simulink model "xyzFuzzyQuadControl"  (R2014b)
settings: Solver=ode45  StartTime=0.0  StopTime=100  RelTol=1e-3
values from neighbouring files (symbols this model uses):
  b = 3.13e-5    (= 3.13e-05)    [Parrametresnnlineaire.m]
  d = 7.50e-7    (= 7.5e-07)    [Parrametresnnlineaire.m]
  g = 9.81    [Parrametresnnlineaire.m]
  Ix = 0.0075    [Parrametresnnlineaire.m]
  Iy = 0.0075    [Parrametresnnlineaire.m]
  Iz = 0.013    [Parrametresnnlineaire.m]
  Jr = 6e-5    (= 6e-05)    [Parrametresnnlineaire.m]
  l = 0.23    [Parrametresnnlineaire.m]
  m = 0.65    [Parrametresnnlineaire.m]
undefined symbols (not defined in the file or in its folder): sigbuilder_block
libraries: fuzblock x6, simulink x5
settings Model: Creator=Khadija  LastModifiedBy=Khadija
settings DataIOCC: LimitDataPoints=off

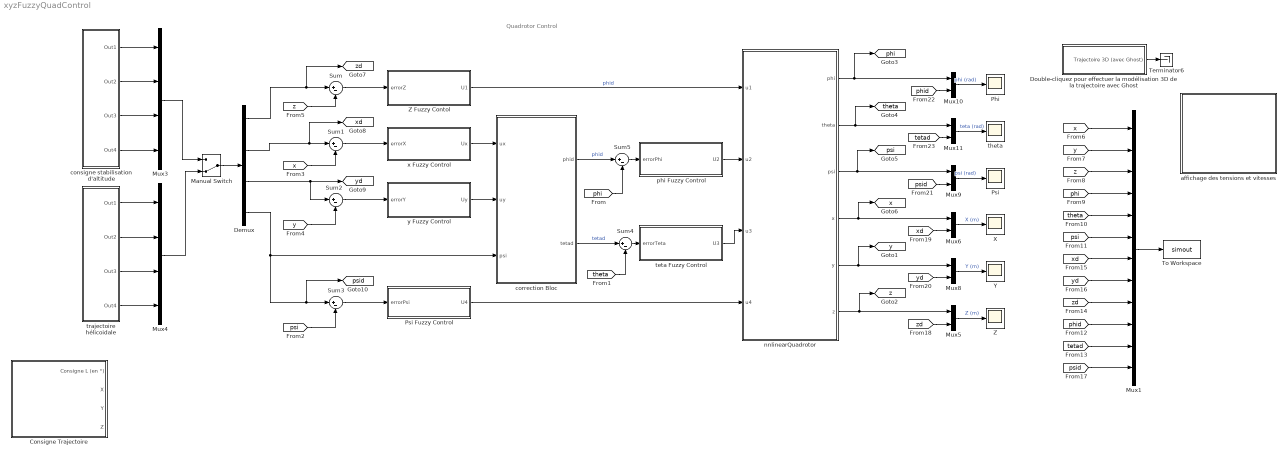
== system xyzFuzzyQuadControl ==
  note: Quadrotor Control
  " Z Fuzzy Contol" : Subsystem
  " phi Fuzzy Control " : Subsystem
  " x Fuzzy Control " : Subsystem
  Consigne Trajectoire : Subsystem  Tag=STV Subsys  LoadFcn=sigbuilder_block('load');  StartFcn=sigbuilder_block('start');  StopFcn=sigbuilder_block('stop');  ClipboardFcn=sigbuilder_block('clipboard');  mask(Sigbuilder block){}
      mask help: Sigbuilder GUI
      mask init:
      | if ~strcmp(get_param(bdroot(gcbh),'SimulationStatus'),'stopped') tuvar = sigbuilder_block('maskInit'); end
      settings: CopyFcn=sigbuilder_block('copy');  DeleteFcn=sigbuilder_block('delete');  ModelCloseFcn=sigbuilder_block('modelClose');  PreSaveFcn=sigbuilder_block('preSave');  PauseFcn=sigbuilder_block('pause')  ContinueFcn=sigbuilder_block('continue')  NameChangeFcn=sigbuilder_block('namechange');  OpenFcn=sigbuilder_block('open',[0 -33.75 864 576.75 ]);  CloseFcn=sigbuilder_block('close');
      mask Display: plot(0,0,100,100,[10,10,40,40,10],[80,20,20,80,80],[40,10],[50,50], [40,27,10],[65,72,56],[40,25,25,10],[28,28,43,43]);
  Demux : Demux
  Double-cliquez pour effectuer la modélisation 3D de la trajectoire avec Ghost : Subsystem
      settings: OpenFcn=trace
  Manual Switch : ManualSwitch  CurrentSetting=0
  Mux1 : Mux  Inputs=12
  Mux{5..6,8..11} (6 alike) : Mux  Inputs=2
  Mux3 : Mux
  Mux4 : Mux
  Phi : Scope
      settings: TimeRange=10  YMin=-0.2  YMax=0.7  SaveName=phi
  Psi : Scope
      settings: TimeRange=10  YMin=0.42  YMax=0.51  SaveName=phi5
  "Psi Fuzzy Control " : Subsystem
  Sum{,1..5} (6 alike) : Sum  Inputs=|+-
  Terminator6 : Terminator
  To Workspace : ToWorkspace  VariableName=simout  SaveFormat=Structure  SampleTime=-1
  X : Scope
      settings: TimeRange=10  YMin=0  YMax=4.5  SaveName=phi4
  Y : Scope
      settings: YMax=4  SaveName=phi2
  "Z " : Scope
      settings: TimeRange=10  YMin=0  YMax=0.45  SaveName=phi9
  affichage des tensions et vitesses : Subsystem
  consigne stabilisation d'altitude : Subsystem
  correction Bloc : Subsystem
  nnlinearQuadrotor : Subsystem
  teta Fuzzy Control : Subsystem
  theta : Scope
      settings: TimeRange=10  YMin=-0.02  YMax=0.16  SaveName=phi1
  trajectoire hélicoidale : Subsystem
  y Fuzzy Control : Subsystem
  tag scope: phi=global, psi=global, psid=global, theta=global, x=global, xd=global, y=global, yd=global, z=global, zd=global
  wires:
  Sum/1 -> " Z Fuzzy Contol"/1(errorZ)
  Sum1/1 -> " x Fuzzy Control "/1(errorX)
  Sum2/1 -> y Fuzzy Control/1(errorY)
  y Fuzzy Control/1("Uy ") -> correction Bloc/2(uy)
  Sum5/1 -> " phi Fuzzy Control "/1(errorPhi)
  Sum3/1 -> "Psi Fuzzy Control "/1(errorPsi)
  nnlinearQuadrotor/2(theta) -> Mux11/1, [theta]
  nnlinearQuadrotor/3(psi) -> Mux9/1, [psi]
  nnlinearQuadrotor/6(z) -> Mux5/1, [z]
  nnlinearQuadrotor/1("phi ") -> Mux10/1, [phi]
  nnlinearQuadrotor/4(x) -> Mux6/1, [x]
  nnlinearQuadrotor/5(y) -> Mux8/1, [y]
  [phi] -> Sum5/2
  [psi] -> Sum3/2
  [z] -> Sum/2
  [x] -> Sum1/2
  [y] -> Sum2/2
  correction Bloc/1(phid) -> Sum5/1  "phid"
  correction Bloc/2(tetad) -> Sum4/1  "tetad"
  Sum4/1 -> teta Fuzzy Control/1(errorTeta)
  [theta] -> Sum4/2
  Mux1/1 -> To Workspace/1
  [phi] -> Mux1/4
  [x] -> Mux1/1
  [y] -> Mux1/2
  [z] -> Mux1/3
  [theta] -> Mux1/5
  [psi] -> Mux1/6
  [psid] -> Mux1/12
  [tetad] -> Mux1/11
  [phid] -> Mux1/10
  [zd] -> Mux1/9
  [yd] -> Mux1/8
  [xd] -> Mux1/7
  Double-cliquez pour effectuer la modélisation 3D de la trajectoire avec Ghost/1(Trajectoire 3D (avec Ghost)) -> Terminator6/1
  Mux5/1 -> "Z "/1  "Z (m)"
  Mux6/1 -> X/1  "X (m)"
  Mux8/1 -> Y/1  "Y (m)"
  Mux9/1 -> Psi/1  "psi (rad)"
  Mux10/1 -> Phi/1  "phi (rad)"
  Mux11/1 -> theta/1  "teta (rad)"
  [psid] -> Mux9/2
  [tetad] -> Mux11/2
  [phid] -> Mux10/2
  [yd] -> Mux8/2
  [zd] -> Mux5/2
  [xd] -> Mux6/2
  Demux/1 -> [zd], Sum/1
  Demux/2 -> [xd], Sum1/1
  Demux/3 -> Sum2/1, [yd]
  Manual Switch/1 -> Demux/1
  Mux3/1 -> Manual Switch/1
  Demux/4 -> correction Bloc/3(psi), [psid], Sum3/1
  " x Fuzzy Control "/1(Ux) -> correction Bloc/1(ux)
  "Psi Fuzzy Control "/1(U4) -> nnlinearQuadrotor/4(u4)
  " phi Fuzzy Control "/1(U2) -> nnlinearQuadrotor/2(u2)
  teta Fuzzy Control/1("U3 ") -> nnlinearQuadrotor/3(u3)
  " Z Fuzzy Contol"/1(U1) -> nnlinearQuadrotor/1(u1)  "phid"
  Mux4/1 -> Manual Switch/2
  trajectoire hélicoidale/1(Out1) -> Mux4/1
  trajectoire hélicoidale/2(Out2) -> Mux4/2
  trajectoire hélicoidale/3(Out3) -> Mux4/3
  trajectoire hélicoidale/4(Out4) -> Mux4/4
  consigne stabilisation d'altitude/1(Out1) -> Mux3/1
  consigne stabilisation d'altitude/2(Out2) -> Mux3/2
  consigne stabilisation d'altitude/3(Out3) -> Mux3/3
  consigne stabilisation d'altitude/4(Out4) -> Mux3/4

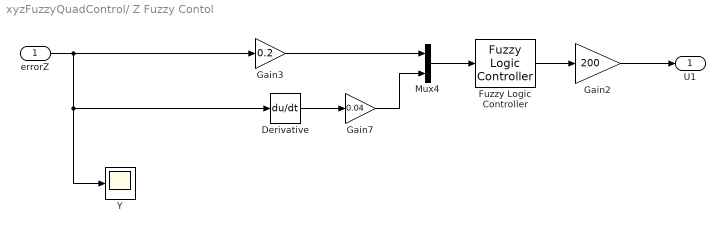
== system xyzFuzzyQuadControl/ Z Fuzzy Contol ==
  errorZ : Inport
  Derivative : Derivative
  Fuzzy Logic Controller : fuzblock/Fuzzy Logic  Controller  fis=ZFLC
  Gain2 : Gain  Gain=200
  Gain3 : Gain  Gain=0.2
  Gain7 : Gain  Gain=0.04
  Mux4 : Mux  Inputs=2
  Y : Scope
      settings: YMin=0  YMax=400  SaveName=phi3
  U1 : Outport
  wires:
  Gain2/1 -> U1/1
  Mux4/1 -> Fuzzy Logic Controller/1
  Gain7/1 -> Mux4/2
  Derivative/1 -> Gain7/1
  Fuzzy Logic Controller/1 -> Gain2/1
  errorZ/1 -> Gain3/1, Y/1, Derivative/1
  Gain3/1 -> Mux4/1

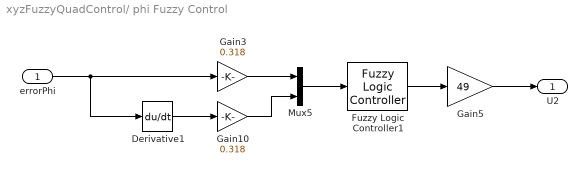
== system xyzFuzzyQuadControl/ phi Fuzzy Control  ==
  errorPhi : Inport
  Derivative1 : Derivative
  Fuzzy Logic Controller1 : fuzblock/Fuzzy Logic  Controller  fis=AngleFLC
  Gain10 : Gain  Gain=0.318
  Gain3 : Gain  Gain=0.318
  Gain5 : Gain  Gain=49
  Mux5 : Mux  Inputs=2
  U2 : Outport
  wires:
  Gain10/1 -> Mux5/2
  Derivative1/1 -> Gain10/1
  Gain3/1 -> Mux5/1
  errorPhi/1 -> Derivative1/1, Gain3/1
  Gain5/1 -> U2/1
  Fuzzy Logic Controller1/1 -> Gain5/1
  Mux5/1 -> Fuzzy Logic Controller1/1

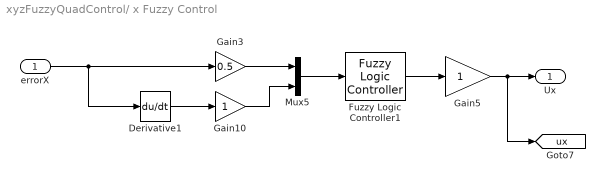
== system xyzFuzzyQuadControl/ x Fuzzy Control  ==
  errorX : Inport
  Derivative1 : Derivative
  Fuzzy Logic Controller1 : fuzblock/Fuzzy Logic  Controller  fis=XYFLC
  Gain10 : Gain
  Gain3 : Gain  Gain=0.5
  Gain5 : Gain
  Mux5 : Mux  Inputs=2
  Ux : Outport
  tag scope: ux=global
  wires:
  Mux5/1 -> Fuzzy Logic Controller1/1
  Fuzzy Logic Controller1/1 -> Gain5/1
  errorX/1 -> Gain3/1, Derivative1/1
  Gain3/1 -> Mux5/1
  Derivative1/1 -> Gain10/1
  Gain10/1 -> Mux5/2
  Gain5/1 -> [ux], Ux/1

== system xyzFuzzyQuadControl/Consigne Trajectoire ==
  Demux : Demux  Tag=STV Demux
  FromWs : FromWorkspace  Tag=STV FromWs  VariableName=tuvar  SampleTime=0
      SigBuilderData=|
      | dataSet.timeRange = [0 100]
      | dataSet.name = 'Group 1'
      | sbobj.Groups.Name = 'Group 1'
      | sbobj.Groups.Signals(1).Name = 'Consigne L (en °)'
      | sbobj.Groups.Signals(1).XData = [0 100]
      | sbobj.Groups.Signals(1).YData = [0 0]
      | sbobj.Groups.Signals(2).Name = 'X'
      | sbobj.Groups.Signals(2).XData = [0 10.05 20 30 40 60 60 70 70 80 90 90 100]
      | sbobj.Groups.Signals(2).YData = [3.9 -3.5 2.15 3.55 -3.5 3.4 3.5 0.5 0.4 -4.2 1.6 1.5 -2.05]
      | sbobj.Groups.Signals(3).Name = 'Y'
      | sbobj.Groups.Signals(3).XData = [0 10 20 30 40 40 50 60 70.1 92 100]
      | sbobj.Groups.Signals(3).YData = [-3.3 3.7 -3.3 -1.8 4.5 4.4 -2.3 -0.4 3.4 -3.4 -3.4]
      | sbobj.Groups.Signals(4).Name = 'Z'
      | sbobj.Groups.Signals(4).XData = [0 10 20 30 40 40 60 72 85 85 100]
      | sbobj.Groups.Signals(4).YData = [5 1.9 3.5 2.3 5.55 5.6 2.4 5 3.7 3.8 1.8]
      | sbobj.Groups.TimeRange = [0 100]
  Consigne L (en °) : Outport  Tag=STV Outport
  X : Outport  Tag=STV Outport  Port=2
  Y : Outport  Tag=STV Outport  Port=3
  Z : Outport  Tag=STV Outport  Port=4
  wires:
  FromWs/1 -> Demux/1
  Demux/1 -> Consigne L (en °)/1
  Demux/2 -> X/1
  Demux/3 -> Y/1
  Demux/4 -> Z/1

== system xyzFuzzyQuadControl/Double-cliquez pour effectuer la modélisation 3D de la trajectoire avec Ghost ==
  Ground : Ground
  Trajectoire 3D (avec Ghost) : Outport
  wires:
  Ground/1 -> Trajectoire 3D (avec Ghost)/1

== system xyzFuzzyQuadControl/Psi Fuzzy Control  ==
  errorPsi : Inport
  Derivative3 : Derivative
  Fuzzy Logic Controller3 : fuzblock/Fuzzy Logic  Controller  fis=AngleFLC
  Gain11 : Gain  Gain=2.36
  Gain6 : Gain  Gain=0.15
  Gain9 : Gain  Gain=0.06
  Mux7 : Mux  Inputs=2
  U4 : Outport
  wires:
  Mux7/1 -> Fuzzy Logic Controller3/1
  Fuzzy Logic Controller3/1 -> Gain11/1
  errorPsi/1 -> Derivative3/1, Gain6/1
  Gain11/1 -> U4/1
  Gain6/1 -> Mux7/1
  Derivative3/1 -> Gain9/1
  Gain9/1 -> Mux7/2

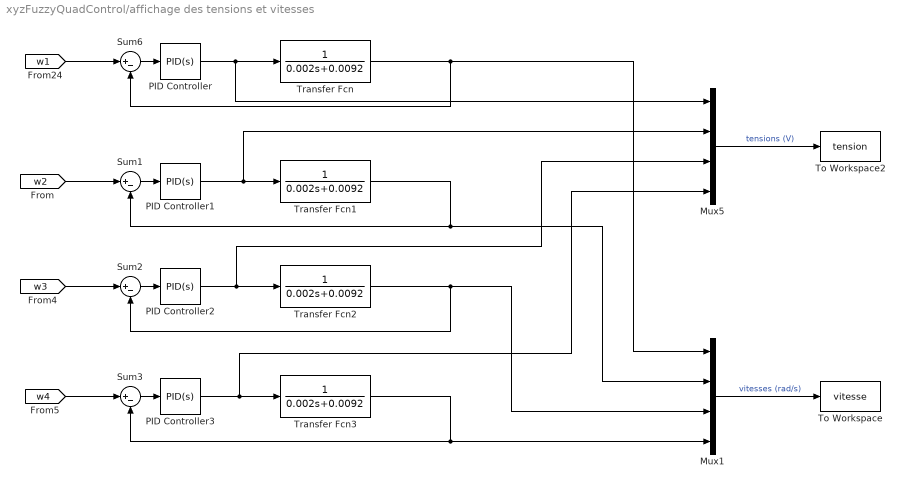
== system xyzFuzzyQuadControl/affichage des tensions et vitesses ==
  Mux1 : Mux
  Mux5 : Mux
  PID Controller{,1..3} (4 alike) : simulink/Continuous/PID Controller  Controller=PID  TimeDomain=Continuous-time  SampleTime=-1  IntegratorMethod=Forward Euler  FilterMethod=Forward Euler  Form=Parallel  P=0.005  I=0.035  D=0  N=100  InitialConditionSource=internal  InitialConditionForIntegrator=0  InitialConditionForFilter=0  ExternalReset=none  LimitOutput=off  UpperSaturationLimit=inf  LowerSaturationLimit=-inf  LinearizeAsGain=on  AntiWindupMode=none  Kb=1  TrackingMode=off  Kt=1  PParamMin=[]  PParamMax=[]  IParamMin=[]  IParamMax=[]  DParamMin=[]  DParamMax=[]  NParamMin=[]  NParamMax=[]  KbParamMin=[]  KbParamMax=[]  KtParamMin=[]  KtParamMax=[]  POutMin=[]  POutMax=[]  IOutMin=[]  IOutMax=[]  DOutMin=[]  DOutMax=[]  NOutMin=[]  NOutMax=[]  KbOutMin=[]  KbOutMax=[]  KtOutMin=[]  KtOutMax=[]  IntegratorOutMin=[]  IntegratorOutMax=[]  FilterOutMin=[]  FilterOutMax=[]  SumOutMin=[]  SumOutMax=[]  SumI1OutMin=[]  SumI1OutMax=[]  SumI2OutMin=[]  SumI2OutMax=[]  SumI3OutMin=[]  SumI3OutMax=[]  SumDOutMin=[]  SumDOutMax=[]  SaturationOutMin=[]  SaturationOutMax=[]  IntegratorContinuousStateAttributes=''  IntegratorStateMustResolveToSignalObject=off  IntegratorRTWStateStorageClass=Auto  FilterContinuousStateAttributes=''  FilterStateMustResolveToSignalObject=off  FilterRTWStateStorageClass=Auto  DifferentiatorICPrevScaledInput=0  DifferentiatorOutMin=[]  DifferentiatorOutMax=[]  UseFilter=on
  Sum{1..3,6} (4 alike) : Sum  Inputs=|+-
  To Workspace : ToWorkspace  VariableName=vitesse  SaveFormat=Structure  SampleTime=-1
  "To Workspace2 " : ToWorkspace  VariableName=tension  SaveFormat=Structure  SampleTime=-1
  Transfer Fcn{,1..3} (4 alike) : TransferFcn  Denominator=[0.002 0.0092]
  wires:
  PID Controller/1 -> Mux5/1, Transfer Fcn/1
  Sum6/1 -> PID Controller/1
  [w1] -> Sum6/1
  Transfer Fcn/1 -> Mux1/1, Sum6/2
  PID Controller1/1 -> Mux5/2, Transfer Fcn1/1
  Sum1/1 -> PID Controller1/1
  [w2] -> Sum1/1
  Transfer Fcn1/1 -> Mux1/2, Sum1/2
  PID Controller2/1 -> Mux5/3, Transfer Fcn2/1
  Sum2/1 -> PID Controller2/1
  [w3] -> Sum2/1
  Transfer Fcn2/1 -> Mux1/3, Sum2/2
  PID Controller3/1 -> Mux5/4, Transfer Fcn3/1
  Sum3/1 -> PID Controller3/1
  [w4] -> Sum3/1
  Transfer Fcn3/1 -> Mux1/4, Sum3/2
  Mux5/1 -> "To Workspace2 "/1  "tensions (V)"
  Mux1/1 -> To Workspace/1  "vitesses (rad/s)"

== system xyzFuzzyQuadControl/consigne stabilisation d'altitude ==
  "Consigne " : Subsystem  Tag=STV Subsys  LoadFcn=sigbuilder_block('load');  StartFcn=sigbuilder_block('start');  StopFcn=sigbuilder_block('stop');  ClipboardFcn=sigbuilder_block('clipboard');  mask(Sigbuilder block){}
      mask help: Sigbuilder GUI
      mask init:
      | if ~strcmp(get_param(bdroot(gcbh),'SimulationStatus'),'stopped') tuvar = sigbuilder_block('maskInit'); end
      settings: CopyFcn=sigbuilder_block('copy');  DeleteFcn=sigbuilder_block('delete');  ModelCloseFcn=sigbuilder_block('modelClose');  PreSaveFcn=sigbuilder_block('preSave');  PauseFcn=sigbuilder_block('pause')  ContinueFcn=sigbuilder_block('continue')  NameChangeFcn=sigbuilder_block('namechange');  OpenFcn=sigbuilder_block('open',[0 -33.75 864 576.75 ]);  CloseFcn=sigbuilder_block('close');
      mask Display: plot(0,0,100,100,[10,10,40,40,10],[80,20,20,80,80],[40,10],[50,50], [40,27,10],[65,72,56],[40,25,25,10],[28,28,43,43]);
  Step2 : Step  SampleTime=0
  Step3 : Step  SampleTime=0
  Step6 : Step  After=0.5  SampleTime=0
  Out1 : Outport
  Out2 : Outport  Port=2
  Out3 : Outport  Port=3
  Out4 : Outport  Port=4
  wires:
  Step6/1 -> Out4/1
  Step3/1 -> Out3/1
  Step2/1 -> Out2/1
  "Consigne "/1(Consigne L (en °)) -> Out1/1

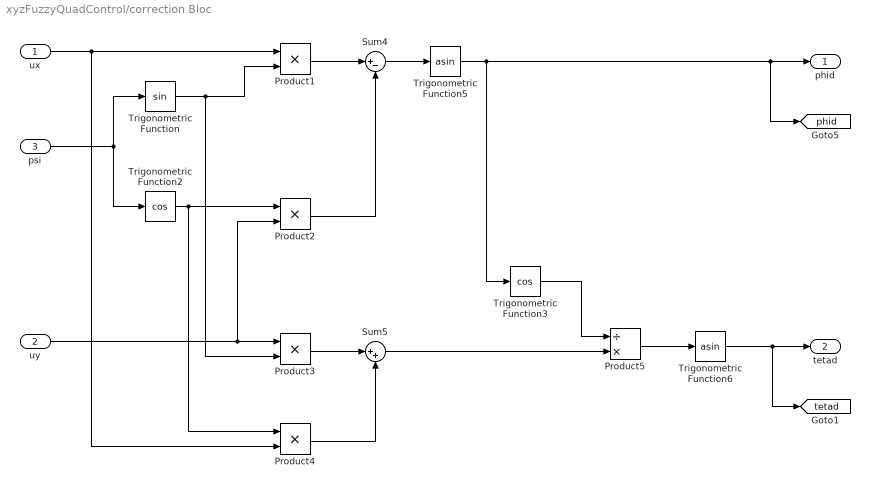
== system xyzFuzzyQuadControl/correction Bloc ==
  ux : Inport
  uy : Inport  Port=2
  psi : Inport  Port=3
  Product{1..4} (4 alike) : Product  Inputs=**
  Product5 : Product  Inputs=/*
  Sum4 : Sum  Inputs=|+-
  Sum5 : Sum  Inputs=|++
  Trigonometric Function : Trigonometry
  Trigonometric Function2 : Trigonometry  Operator=cos
  Trigonometric Function3 : Trigonometry  Operator=cos
  Trigonometric Function5 : Trigonometry  Operator=asin
  Trigonometric Function6 : Trigonometry  Operator=asin
  phid : Outport
  tetad : Outport  Port=2
  tag scope: phid=global, tetad=global
  wires:
  Trigonometric Function3/1 -> Product5/1
  Product2/1 -> Sum4/2
  ux/1 -> Product1/1, Product4/2
  Sum5/1 -> Product5/2
  psi/1 -> Trigonometric Function/1, Trigonometric Function2/1
  Trigonometric Function/1 -> Product3/2, Product1/2
  Product1/1 -> Sum4/1
  Trigonometric Function2/1 -> Product4/1, Product2/1
  Sum4/1 -> Trigonometric Function5/1
  Product4/1 -> Sum5/2
  Product3/1 -> Sum5/1
  Product5/1 -> Trigonometric Function6/1
  uy/1 -> Product2/2, Product3/1
  Trigonometric Function5/1 -> [phid], phid/1, Trigonometric Function3/1
  Trigonometric Function6/1 -> [tetad], tetad/1

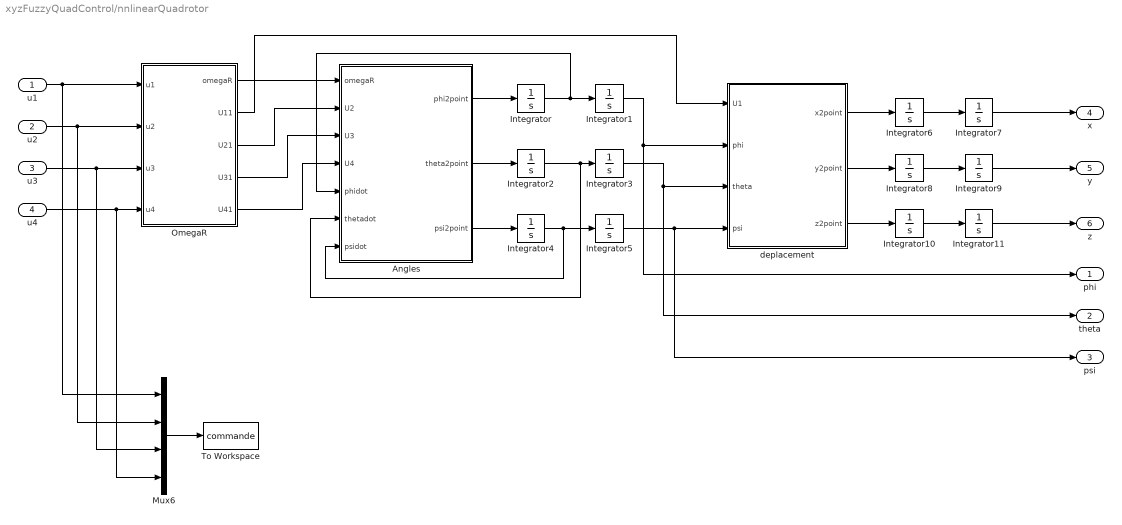
== system xyzFuzzyQuadControl/nnlinearQuadrotor ==
  u1 : Inport
  u2 : Inport  Port=2
  u3 : Inport  Port=3
  u4 : Inport  Port=4
  Angles : Subsystem
  Integrator : Integrator  UpperSaturationLimit=0.5  LowerSaturationLimit=-0.5
  Integrator{1,3,5,7,9,11} (6 alike) : Integrator
  Integrator10 : Integrator  UpperSaturationLimit=1  LowerSaturationLimit=-1
  Integrator2 : Integrator  UpperSaturationLimit=0.5  LowerSaturationLimit=-0.5
  Integrator4 : Integrator  UpperSaturationLimit=0.5  LowerSaturationLimit=-0.5
  Integrator6 : Integrator  UpperSaturationLimit=1  LowerSaturationLimit=-1
  Integrator8 : Integrator  UpperSaturationLimit=1  LowerSaturationLimit=-1
  Mux6 : Mux
  OmegaR : Subsystem
  To Workspace : ToWorkspace  VariableName=commande  SaveFormat=Structure  SampleTime=-1
  deplacement : Subsystem
  "phi " : Outport
  theta : Outport  Port=2
  psi : Outport  Port=3
  x : Outport  Port=4
  y : Outport  Port=5
  z : Outport  Port=6
  wires:
  u1/1 -> Mux6/1, OmegaR/1(u1)
  u4/1 -> Mux6/4, OmegaR/4(u4)
  u2/1 -> Mux6/2, OmegaR/2(u2)
  u3/1 -> Mux6/3, OmegaR/3(u3)
  Integrator10/1 -> Integrator11/1
  Integrator8/1 -> Integrator9/1
  Integrator6/1 -> Integrator7/1
  Integrator7/1 -> x/1
  OmegaR/2("U11 ") -> deplacement/1(U1)
  deplacement/3(z2point) -> Integrator10/1
  deplacement/1(x2point) -> Integrator6/1
  Integrator9/1 -> y/1
  deplacement/2(y2point) -> Integrator8/1
  Integrator2/1 -> Angles/6(thetadot), Integrator3/1
  Integrator4/1 -> Angles/7(psidot), Integrator5/1
  Integrator3/1 -> deplacement/3(theta), theta/1
  Angles/2(theta2point) -> Integrator2/1
  Angles/3(psi2point) -> Integrator4/1
  Angles/1("phi2point ") -> Integrator/1
  Integrator/1 -> Angles/5(phidot), Integrator1/1
  Integrator1/1 -> "phi "/1, deplacement/2(phi)
  OmegaR/4(U31) -> Angles/3(U3)
  OmegaR/1(omegaR) -> Angles/1(omegaR)
  OmegaR/3(U21) -> Angles/2(U2)
  OmegaR/5(U41) -> Angles/4("U4 ")
  Integrator11/1 -> z/1
  Integrator5/1 -> psi/1, deplacement/4(psi)
  Mux6/1 -> To Workspace/1

== system xyzFuzzyQuadControl/teta Fuzzy Control ==
  errorTeta : Inport
  Derivative2 : Derivative
  Fuzzy Logic Controller2 : fuzblock/Fuzzy Logic  Controller  fis=AngleFLC
  Gain12 : Gain  Gain=0.318
  Gain4 : Gain  Gain=0.318
  Gain8 : Gain  Gain=49
  Mux6 : Mux  Inputs=2
  "U3 " : Outport
  wires:
  Gain8/1 -> "U3 "/1
  Fuzzy Logic Controller2/1 -> Gain8/1
  errorTeta/1 -> Derivative2/1, Gain4/1
  Gain4/1 -> Mux6/1
  Mux6/1 -> Fuzzy Logic Controller2/1
  Gain12/1 -> Mux6/2
  Derivative2/1 -> Gain12/1

== system xyzFuzzyQuadControl/trajectoire hélicoidale ==
  Ramp : simulink/Sources/Ramp  slope=0.1  start=0  X0=0
  Sine Wave1 : Sin  Amplitude=4  Frequency=0.25  SampleTime=0
  Sine Wave2 : Sin  Amplitude=4  Frequency=0.25  Phase=3.14/2  SampleTime=0
  Step1 : Step  After=0.5  SampleTime=0
  Out1 : Outport
  Out2 : Outport  Port=2
  Out3 : Outport  Port=3
  Out4 : Outport  Port=4
  wires:
  Sine Wave1/1 -> Out2/1
  Sine Wave2/1 -> Out3/1
  Step1/1 -> Out4/1
  Ramp/1 -> Out1/1

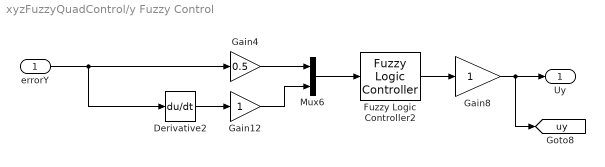
== system xyzFuzzyQuadControl/y Fuzzy Control ==
  errorY : Inport
  Derivative2 : Derivative
  Fuzzy Logic Controller2 : fuzblock/Fuzzy Logic  Controller  fis=XYFLC
  Gain12 : Gain
  Gain4 : Gain  Gain=0.5
  Gain8 : Gain
  Mux6 : Mux  Inputs=2
  "Uy " : Outport
  tag scope: uy=global
  wires:
  Fuzzy Logic Controller2/1 -> Gain8/1
  errorY/1 -> Derivative2/1, Gain4/1
  Gain4/1 -> Mux6/1
  Mux6/1 -> Fuzzy Logic Controller2/1
  Gain12/1 -> Mux6/2
  Derivative2/1 -> Gain12/1
  Gain8/1 -> [uy], "Uy "/1

== system xyzFuzzyQuadControl/consigne stabilisation d'altitude/Consigne  ==
  Demux : Demux  Tag=STV Demux  Outputs=1
  FromWs : FromWorkspace  Tag=STV FromWs  VariableName=tuvar  SampleTime=0
      SigBuilderData=|
      | dataSet.timeRange = [0 20]
      | dataSet.name = 'Group 1'
      | sbobj.Groups.Name = 'Group 1'
      | sbobj.Groups.Signals.Name = 'Consigne L (en °)'
      | sbobj.Groups.Signals.XData = [0 1 1 10 10 20]
      | sbobj.Groups.Signals.YData = [0 0 1 1 2 2]
      | sbobj.Groups.TimeRange = [0 20]
  Consigne L (en °) : Outport  Tag=STV Outport
  wires:
  FromWs/1 -> Demux/1
  Demux/1 -> Consigne L (en °)/1

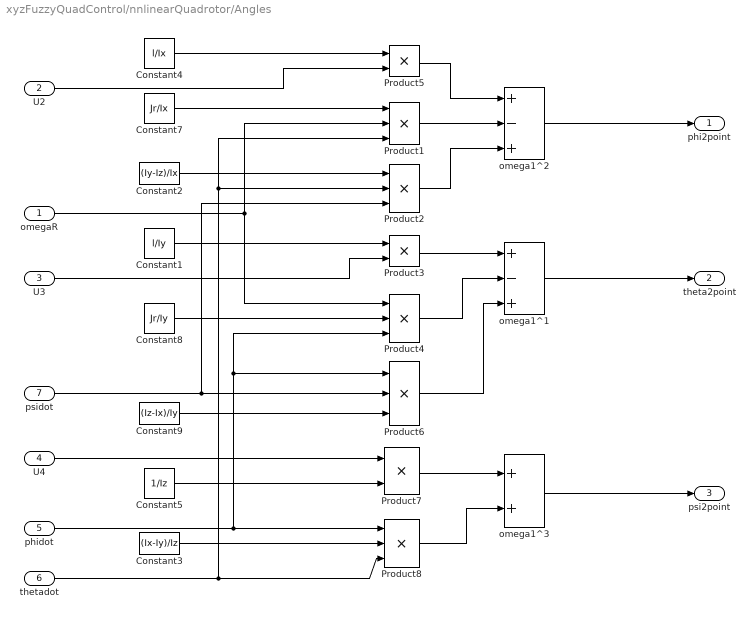
== system xyzFuzzyQuadControl/nnlinearQuadrotor/Angles ==
  omegaR : Inport
  U2 : Inport  Port=2
  U3 : Inport  Port=3
  "U4 " : Inport  Port=4
  phidot : Inport  Port=5
  thetadot : Inport  Port=6
  psidot : Inport  Port=7
  Constant1 : Constant  Value=l/Iy
  Constant2 : Constant  Value=(Iy-Iz)/Ix
  Constant3 : Constant  Value=(Ix-Iy)/Iz
  Constant4 : Constant  Value=l/Ix
  Constant5 : Constant  Value=1/Iz
  Constant7 : Constant  Value=Jr/Ix
  Constant8 : Constant  Value=Jr/Iy
  Constant9 : Constant  Value=(Iz-Ix)/Iy
  Product{1..2,4,6,8} (5 alike) : Product  Inputs=***
  Product3 : Product  Inputs=**
  Product5 : Product  Inputs=**
  Product7 : Product  Inputs=**
  omega1^1 : Sum  Inputs=+-+
  omega1^2 : Sum  Inputs=+-+
  omega1^3 : Sum
  "phi2point " : Outport
  theta2point : Outport  Port=2
  psi2point : Outport  Port=3
  wires:
  Constant2/1 -> Product2/1
  Constant4/1 -> Product5/1
  Constant7/1 -> Product1/1
  omegaR/1 -> Product4/1, Product1/2
  U2/1 -> Product5/2
  U3/1 -> Product3/2
  Constant9/1 -> Product6/3
  psidot/1 -> Product2/3, Product6/2
  thetadot/1 -> Product1/3, Product2/2, Product8/3
  phidot/1 -> Product4/3, Product6/1, Product8/1
  Product1/1 -> omega1^2/2
  Constant1/1 -> Product3/1
  Product7/1 -> omega1^3/1
  Product3/1 -> omega1^1/1
  Constant8/1 -> Product4/2
  Product6/1 -> omega1^1/3
  Product5/1 -> omega1^2/1
  Product2/1 -> omega1^2/3
  Product4/1 -> omega1^1/2
  omega1^2/1 -> "phi2point "/1
  omega1^1/1 -> theta2point/1
  omega1^3/1 -> psi2point/1
  Constant5/1 -> Product7/2
  "U4 "/1 -> Product7/1
  Product8/1 -> omega1^3/2
  Constant3/1 -> Product8/2

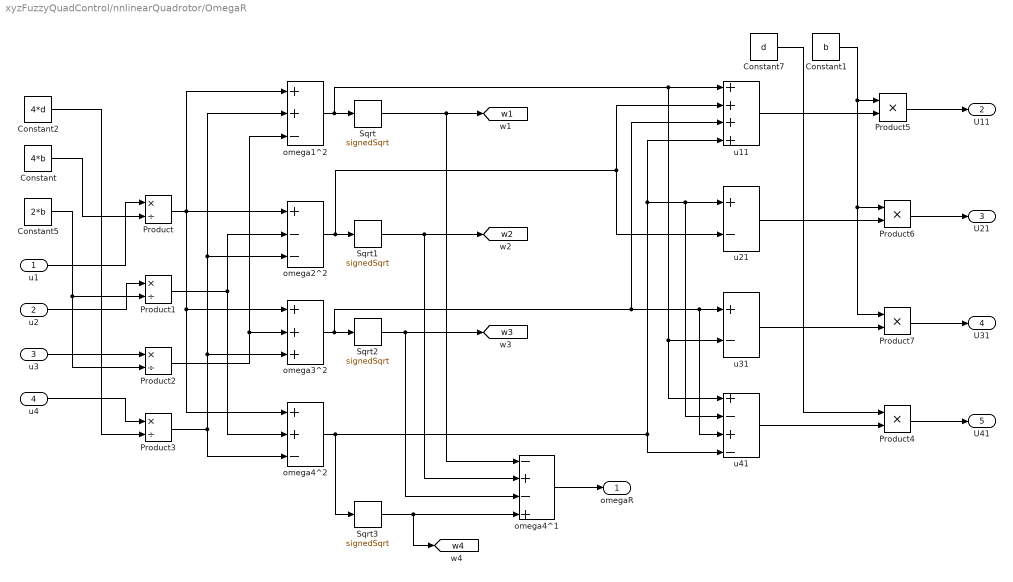
== system xyzFuzzyQuadControl/nnlinearQuadrotor/OmegaR ==
  u1 : Inport
  u2 : Inport  Port=2
  u3 : Inport  Port=3
  u4 : Inport  Port=4
  Constant : Constant  Value=4*b
  Constant1 : Constant  Value=b
  Constant2 : Constant  Value=4*d
  Constant5 : Constant  Value=2*b
  Constant7 : Constant  Value=d
  Product{,1..3} (4 alike) : Product  Inputs=*/
  Product{4..7} (4 alike) : Product  Inputs=**
  Sqrt{,1..3} (4 alike) : Sqrt  Operator=signedSqrt  OutputSignalType=real  SaturateOnIntegerOverflow=on
  omega1^2 : Sum  Inputs=++-
  omega2^2 : Sum  Inputs=+--
  omega3^2 : Sum  Inputs=+++
  omega4^1 : Sum  Inputs=-+-+
  omega4^2 : Sum  Inputs=++-
  u11 : Sum  Inputs=++++
  u21 : Sum  Inputs=+-
  u31 : Sum  Inputs=+-
  "u41 " : Sum  Inputs=+-+-
  omegaR : Outport
  "U11 " : Outport  Port=2
  U21 : Outport  Port=3
  U31 : Outport  Port=4
  U41 : Outport  Port=5
  tag scope: w1=global, w2=global, w3=global, w4=global
  wires:
  u11/1 -> Product5/2
  Product5/1 -> "U11 "/1
  Product7/1 -> U31/1
  omega4^2/1 -> "u41 "/4, u11/4, u21/1, "u41 "/2, Sqrt3/1
  Product1/1 -> omega2^2/2, omega4^2/2
  Product6/1 -> U21/1
  omega2^2/1 -> Sqrt1/1, u21/2, u11/2
  Sqrt3/1 -> [w4], omega4^1/4
  Product2/1 -> omega3^2/2, omega1^2/3
  Constant5/1 -> Product2/2, Product1/2
  omega1^2/1 -> Sqrt/1, u11/1, u31/2, "u41 "/1
  Sqrt1/1 -> [w2], omega4^1/2
  Product4/1 -> U41/1
  u31/1 -> Product7/2
  u21/1 -> Product6/2
  Constant/1 -> Product/2
  u3/1 -> Product2/1
  Product3/1 -> omega4^2/3, omega3^2/3, omega2^2/3, omega1^2/2
  u4/1 -> Product3/1
  Constant1/1 -> Product7/1, Product6/1, Product5/1
  "u41 "/1 -> Product4/2
  u1/1 -> Product/1
  Sqrt2/1 -> omega4^1/3, [w3]
  Constant2/1 -> Product3/2
  Constant7/1 -> Product4/1
  Product/1 -> omega2^2/1, omega3^2/1, omega4^2/1, omega1^2/1
  u2/1 -> Product1/1
  omega3^2/1 -> Sqrt2/1, u11/3, "u41 "/3, u31/1
  omega4^1/1 -> omegaR/1
  Sqrt/1 -> [w1], omega4^1/1

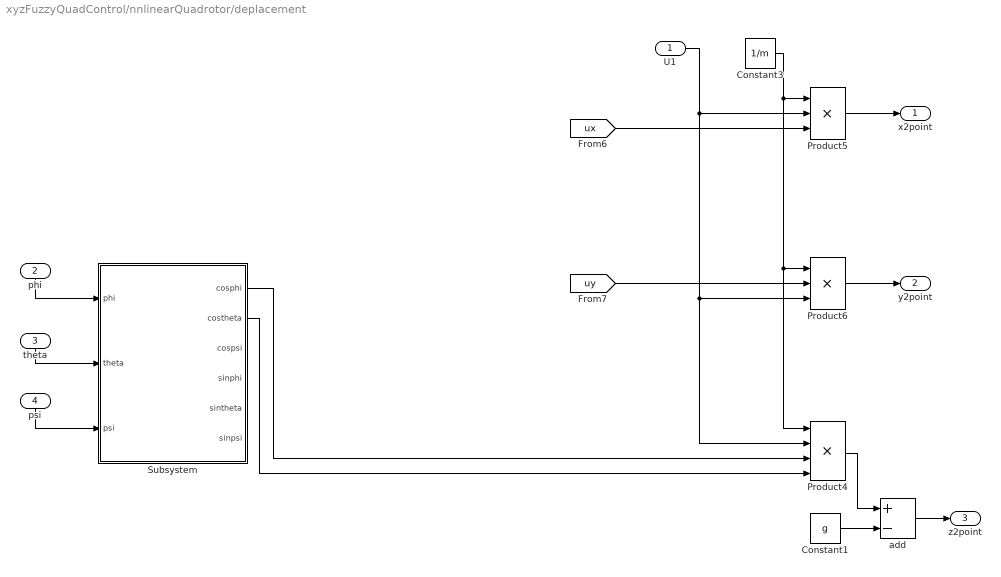
== system xyzFuzzyQuadControl/nnlinearQuadrotor/deplacement ==
  U1 : Inport
  phi : Inport  Port=2
  theta : Inport  Port=3
  psi : Inport  Port=4
  Constant1 : Constant  Value=g
  Constant3 : Constant  Value=1/m
  Product4 : Product  Inputs=****
  Product5 : Product  Inputs=***
  Product6 : Product  Inputs=***
  Subsystem : Subsystem
  add : Sum  Inputs=+-
  x2point : Outport
  y2point : Outport  Port=2
  z2point : Outport  Port=3
  wires:
  Product4/1 -> add/1
  Product6/1 -> y2point/1
  U1/1 -> Product5/2, Product6/3, Product4/2
  add/1 -> z2point/1
  Constant3/1 -> Product5/1, Product4/1, Product6/1
  Product5/1 -> x2point/1
  Constant1/1 -> add/2
  phi/1 -> Subsystem/1(phi)
  theta/1 -> Subsystem/2(theta)
  psi/1 -> Subsystem/3(psi)
  Subsystem/1(cosphi) -> Product4/3
  Subsystem/2(costheta) -> Product4/4
  [ux] -> Product5/3
  [uy] -> Product6/2

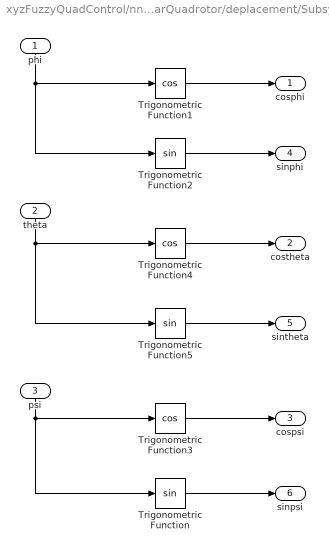
== system xyzFuzzyQuadControl/nnlinearQuadrotor/deplacement/Subsystem ==
  phi : Inport
  theta : Inport  Port=2
  psi : Inport  Port=3
  Trigonometric Function : Trigonometry
  Trigonometric Function1 : Trigonometry  Operator=cos
  Trigonometric Function2 : Trigonometry
  Trigonometric Function3 : Trigonometry  Operator=cos
  Trigonometric Function4 : Trigonometry  Operator=cos
  Trigonometric Function5 : Trigonometry
  cosphi : Outport
  costheta : Outport  Port=2
  cospsi : Outport  Port=3
  sinphi : Outport  Port=4
  sintheta : Outport  Port=5
  sinpsi : Outport  Port=6
  wires:
  Trigonometric Function2/1 -> sinphi/1
  psi/1 -> Trigonometric Function3/1, Trigonometric Function/1
  phi/1 -> Trigonometric Function2/1, Trigonometric Function1/1
  theta/1 -> Trigonometric Function5/1, Trigonometric Function4/1
  Trigonometric Function5/1 -> sintheta/1
  Trigonometric Function/1 -> sinpsi/1
  Trigonometric Function3/1 -> cospsi/1
  Trigonometric Function1/1 -> cosphi/1
  Trigonometric Function4/1 -> costheta/1
